simulink model "firBench_cValidation"  (R2017b)
settings: Solver=FixedStepDiscrete  StartTime=0.0  StopTime=10000  FixedStep=0.1  RelTol=1e-3
libraries: dspsrcs4 x1
settings Model: Creator=cyarp  LastModifiedBy=cyarp

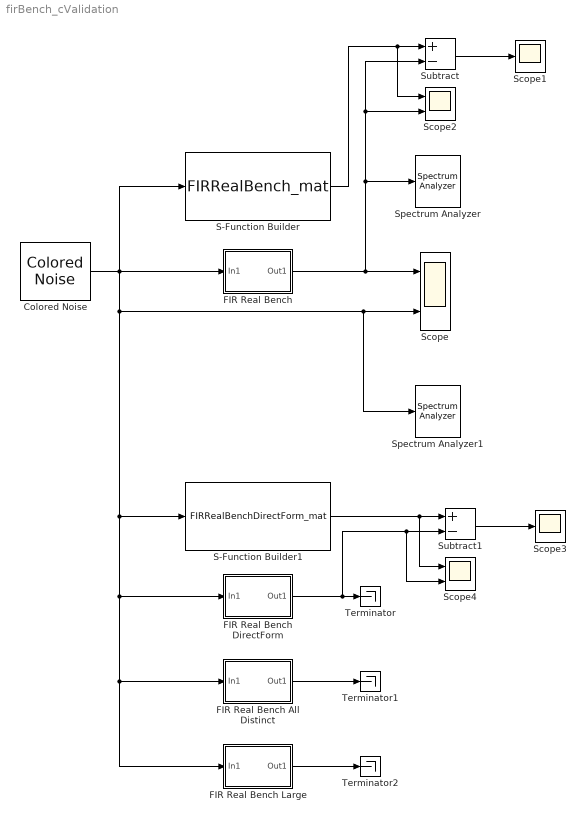
== system firBench_cValidation ==
  Colored Noise : dspsrcs4/Colored Noise  Color=white  InverseFrequencyPower=1  NumChannels=1  OutputDataType=single  SamplesPerFrame=1  SampleTime=1  RandomStream=mt19937ar with seed  Seed=67  SimulateUsing=Interpreted execution
      settings: SourceProductName=DSP System Toolbox  SourceProductBaseCode=DS
  FIR Real Bench : Subsystem
  FIR Real Bench All Distinct : Subsystem
  FIR Real Bench DirectForm : Subsystem
  FIR Real Bench Large : Subsystem
  S-Function Builder : S-Function  InitFcn=try, set_param(gcb,'FunctionName','FIRRealBench_mat'), end  FunctionName=FIRRealBench_mat  SFunctionModules=FIRRealBench_mat_wrapper FIRRealBench  SFunctionDeploymentMode=off  EnableBusSupport=off  mask(S-Function Builder){}
      mask help: Simulink:masks:SFunctionBuilder_MD
      mask init:
      | val = [[.9  0.75 0.75 1 1 .9 .9 1]',[1 1 0.75 0.75 .9 .9 1 .9]'];try , sys = get_param(gcb,'SfunBuilderFcnName');if isempty(sys), sys = get_param(gcb,'FunctionName'); end,catch, sys = get_param(gcb,'FunctionName'); end
      settings: CopyFcn=set_param(gcbh,'LinkStatus','none')  PreSaveFcn=try, set_param(gcb,'FunctionName','FIRRealBench_mat'), end  OpenFcn=sfunctionwizard(gcbh)
      mask Display: plot(val(:,1),val(:,2)),disp(sys), port_label('input',1,'In1'), port_label('output',1,'Out1')
  S-Function Builder1 : S-Function  InitFcn=try, set_param(gcb,'FunctionName','FIRRealBenchDirectForm_mat'), end  FunctionName=FIRRealBenchDirectForm_mat  SFunctionModules=FIRRealBenchDirectForm_mat_wrapper FIRRealBenchDirectForm  SFunctionDeploymentMode=off  EnableBusSupport=off  mask(S-Function Builder){}
      mask help: Simulink:masks:SFunctionBuilder_MD
      mask init: same as firBench_cValidation/S-Function Builder
      settings: CopyFcn=set_param(gcbh,'LinkStatus','none')  PreSaveFcn=try, set_param(gcb,'FunctionName','FIRRealBenchDirectForm_mat'), end  OpenFcn=sfunctionwizard(gcbh)
      mask Display: plot(val(:,1),val(:,2)),disp(sys), port_label('input',1,'In1'), port_label('output',1,'Out1')
  Scope : Scope  NumInputPorts=2
  Scope1 : Scope
  Scope2 : Scope  NumInputPorts=2
  Scope3 : Scope
  Scope4 : Scope  NumInputPorts=2
  Spectrum Analyzer : SpectrumAnalyzer
  Spectrum Analyzer1 : SpectrumAnalyzer
  Subtract : Sum  Inputs=+-
  Subtract1 : Sum  Inputs=+-
  Terminator : Terminator
  Terminator1 : Terminator
  Terminator2 : Terminator
  wires:
  FIR Real Bench/1(Out1) -> Subtract/2, Scope2/2, Spectrum Analyzer/1, Scope/1
  FIR Real Bench DirectForm/1(Out1) -> Scope4/2, Subtract1/2, Terminator/1
  Colored Noise/1 -> S-Function Builder/1, FIR Real Bench/1(In1), S-Function Builder1/1, FIR Real Bench Large/1(In1), FIR Real Bench All Distinct/1(In1), FIR Real Bench DirectForm/1(In1), Spectrum Analyzer1/1, Scope/2
  FIR Real Bench All Distinct/1(Out1) -> Terminator1/1
  FIR Real Bench Large/1(Out1) -> Terminator2/1
  Subtract/1 -> Scope1/1
  S-Function Builder/1 -> Scope2/1, Subtract/1
  Subtract1/1 -> Scope3/1
  S-Function Builder1/1 -> Scope4/1, Subtract1/1

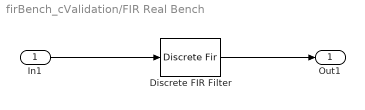
== system firBench_cValidation/FIR Real Bench ==
  In1 : Inport
  Discrete FIR Filter : DiscreteFir  FilterStructure=Direct form transposed  Coefficients=[0.4, 0.2, 0.04, 0.1, 0.4, 0.2, 0.04, 0.1]  InitialStates=[0, 1, 0, 0, 0, 0, 0]
  Out1 : Outport
  wires:
  Discrete FIR Filter/1 -> Out1/1
  In1/1 -> Discrete FIR Filter/1

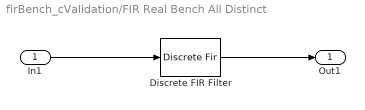
== system firBench_cValidation/FIR Real Bench All Distinct ==
  In1 : Inport
  Discrete FIR Filter : DiscreteFir  FilterStructure=Direct form transposed  Coefficients=(1:1:8)+1
  Out1 : Outport
  wires:
  Discrete FIR Filter/1 -> Out1/1
  In1/1 -> Discrete FIR Filter/1

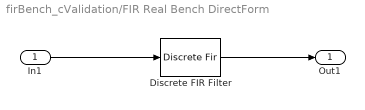
== system firBench_cValidation/FIR Real Bench DirectForm ==
  In1 : Inport
  Discrete FIR Filter : DiscreteFir  Coefficients=[0.4, 0.2, 0.04, 0.1, 0.4, 0.2, 0.04, 0.1]  InitialStates=[0, 1, 0, 0, 0, 0, 0]
  Out1 : Outport
  wires:
  Discrete FIR Filter/1 -> Out1/1
  In1/1 -> Discrete FIR Filter/1

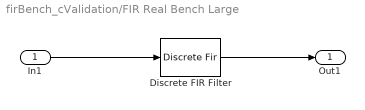
== system firBench_cValidation/FIR Real Bench Large ==
  In1 : Inport
  Discrete FIR Filter : DiscreteFir  FilterStructure=Direct form transposed  Coefficients=(1:1:128)+1
  Out1 : Outport
  wires:
  Discrete FIR Filter/1 -> Out1/1
  In1/1 -> Discrete FIR Filter/1
